simulink model "fstTest"  (R2016b)
settings: Solver=VariableStepAuto  StartTime=0.0  StopTime=10.0  RelTol=1e-3
libraries: simulink x1
settings Model: Creator=lenovo  LastModifiedBy=lenovo

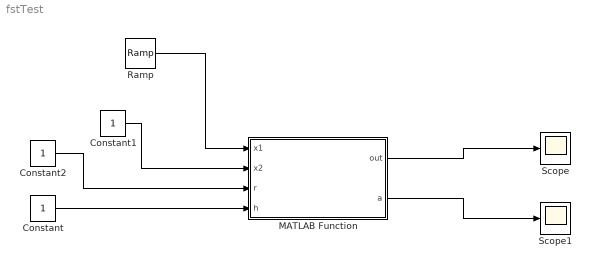
== system fstTest ==
  Constant : Constant
  Constant1 : Constant
  Constant2 : Constant
  MATLAB Function : MATLAB Function  TreatAsAtomicUnit=on
  Ramp : simulink/Sources/Ramp  slope=1  start=0  X0=0
  Scope : Scope
  Scope1 : Scope
  wires:
  Constant/1 -> MATLAB Function/4(h)
  Constant2/1 -> MATLAB Function/3(r)
  Constant1/1 -> MATLAB Function/2(x2)
  Ramp/1 -> MATLAB Function/1(x1)
  MATLAB Function/1(out) -> Scope/1
  MATLAB Function/2(a) -> Scope1/1

== matlab function fstTest/MATLAB Function ==
  data: x1 input; out output; x2 input; r input; h input; a output
function [out,a] = fst_test(x1,x2,r,h)
d=r*h;
d0=d*h;
y=x1+h*x2;
a0=sqrt(d*d+8*r*abs(y));
if abs(y)>d0
    a=x2+0.5*a0-0.5*d;
else
    a=x2+y/h;
end
if abs(a)<=d
    out=-r*a/d;
else
    out=-r*sign(a);
end

end
